simulink model "BLAC_MotorCtrl_Math"  (R2025b)
settings: Solver=FixedStepDiscrete  StartTime=0.0  StopTime=5  FixedStep=MC_Sim_BaseStep  RelTol=1e-3  EnableMultiTasking=on
values from neighbouring files (symbols this model uses):
  MC_Hardware_Chip_ADCResultBit = 0.0    [MotorControlDataDictionary_Math.sldd]
  MC_Hardware_Chip_ADCVoltageMax = 1.0    [MotorControlDataDictionary_Math.sldd]
  MC_Hardware_Chip_ADCVoltageRefence = 0.0    [MotorControlDataDictionary_Math.sldd]
  MC_Hardware_Chip_CSAGain = 1.0    [MotorControlDataDictionary_Math.sldd]
  MC_Sim_BaseStep = 2.5E-8    [MotorControlDataDictionary_Math.sldd]
  MC_Sim_HFTStep = 6.6675E-5    [MotorControlDataDictionary_Math.sldd]
undefined symbols (not defined in the file or in its folder): MC_MOS_DeadTime, MC_Motor_Phi, MC_Motor_Rotor_Pn, MC_Motor_Stator_Ld, MC_Motor_Stator_Lq, MC_Motor_Stator_Rs, MC_Param_CurrentPI_Ki, MC_Param_CurrentPI_Kp, MC_Param_CurrentPI_UdInteMax, MC_Param_CurrentPI_UdInteMin, MC_Param_CurrentPI_UdMax, MC_Param_CurrentPI_UdMin, MC_Param_CurrentPI_UqInteMax, MC_Param_CurrentPI_UqInteMin, MC_Param_CurrentPI_UqMax, MC_Param_CurrentPI_UqMin, MC_Param_Flux_Gamma, MC_Param_Flux_Lalpha, MC_Param_Flux_Lbeta, MC_Param_Flux_Ralpha, MC_Param_Flux_Rbeta, MC_Param_Luen_BEMFalpha, MC_Param_Luen_BEMFbeta, MC_Param_Luen_BEMFErr, MC_Param_Luen_Currentalpha, MC_Param_Luen_Currentbeta, MC_Param_Luen_CurrentErr, MC_Param_Luen_PLL_Ki, MC_Param_Luen_PLL_Kp, MC_Param_Luen_Voltagealpha, MC_Param_Luen_Voltagebeta, MC_Param_PhasetoReal, MC_Param_SMO_CoffA, MC_Param_SMO_CoffB, MC_Param_SpeedtoTheta, MC_Param_SVPWM_DutyMax, MC_Param_SVPWM_DutyMin, MC_Param_SVPWM_SampleOffset1, MC_Param_SVPWM_SampleOffset2, MC_Param_SVPWM_SampleValid
libraries: simulink x31, nesl_utility x22, ee_lib x21, fl_lib x16, spsSeriesRLCBranchLib x2, spsVoltageMeasurementLib x2
(part 2 of 5)

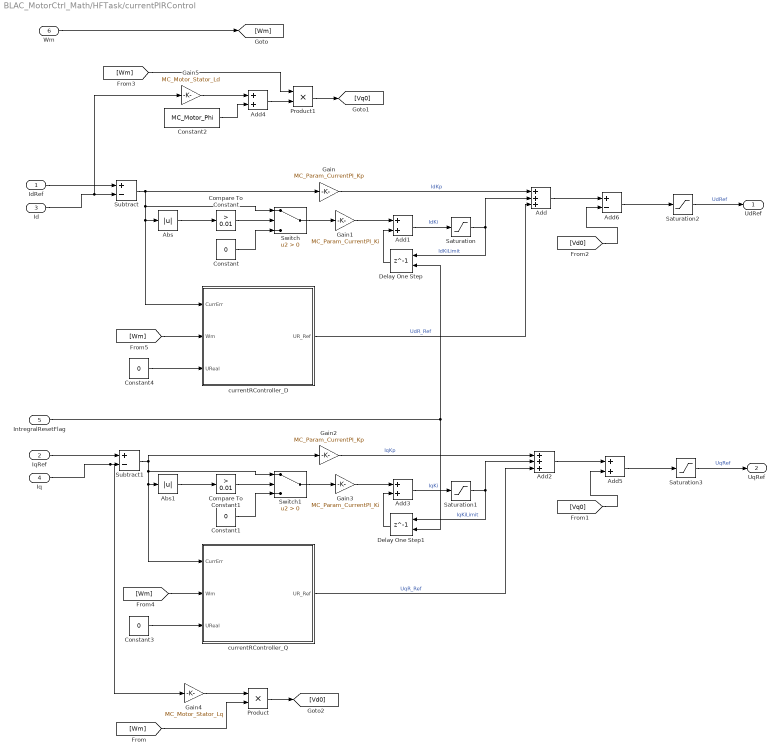
== system BLAC_MotorCtrl_Math/HFTask/currentPIRControl ==
  IdRef : Inport
  IqRef : Inport  Port=2
  Id : Inport  Port=3
  Iq : Inport  Port=4
  IntregralResetFlag : Inport  Port=5
  Wm : Inport  Port=6
  Abs : Abs  SaturateOnIntegerOverflow=off
  Abs1 : Abs  SaturateOnIntegerOverflow=off
  Add : Sum  Inputs=+++
  Add1 : Sum  OutDataTypeStr=single
  Add2 : Sum  Inputs=+++
  Add3 : Sum  OutDataTypeStr=single
  Add4 : Sum
  Add5 : Sum
  Add6 : Sum  Inputs=+-
  Compare To Constant : simulink/Logic and Bit Operations/Compare To Constant  relop=>  const=0.01  OutDataTypeStr=boolean
  Compare To Constant1 : simulink/Logic and Bit Operations/Compare To Constant  relop=>  const=0.01  OutDataTypeStr=boolean
  Constant{,1,3..4} (4 alike) : Constant  Value=0  OutDataTypeStr=single
  Constant2 : Constant  Value=MC_Motor_Phi  OutDataTypeStr=single
  Delay One Step : Delay  DelayLength=1  ExternalReset=Level
      settings: InputPortMap=u0,r5
  Delay One Step1 : Delay  DelayLength=1  ExternalReset=Level
      settings: InputPortMap=u0,r5
  Gain : Gain  Gain=MC_Param_CurrentPI_Kp  OutDataTypeStr=single
  Gain1 : Gain  Gain=MC_Param_CurrentPI_Ki  OutDataTypeStr=single
  Gain2 : Gain  Gain=MC_Param_CurrentPI_Kp  OutDataTypeStr=single
  Gain3 : Gain  Gain=MC_Param_CurrentPI_Ki  OutDataTypeStr=single
  Gain4 : Gain  Gain=MC_Motor_Stator_Lq
  Gain5 : Gain  Gain=MC_Motor_Stator_Ld
  Product : Product
  Product1 : Product
  Saturation : Saturate  UpperLimit=MC_Param_CurrentPI_UdInteMax  LowerLimit=MC_Param_CurrentPI_UdInteMin
  Saturation1 : Saturate  UpperLimit=MC_Param_CurrentPI_UqInteMax  LowerLimit=MC_Param_CurrentPI_UqInteMin
  Saturation2 : Saturate  UpperLimit=MC_Param_CurrentPI_UdMax  LowerLimit=MC_Param_CurrentPI_UdMin
  Saturation3 : Saturate  UpperLimit=MC_Param_CurrentPI_UqMax  LowerLimit=MC_Param_CurrentPI_UqMin
  Subtract : Sum  Inputs=+-
  Subtract1 : Sum  Inputs=+-
  Switch : Switch  Criteria=u2 > Threshold  SaturateOnIntegerOverflow=off  InputSameDT=off
  Switch1 : Switch  Criteria=u2 > Threshold  SaturateOnIntegerOverflow=off  InputSameDT=off
  currentRController_D : Subsystem
  currentRController_Q : Subsystem
  UdRef : Outport
  UqRef : Outport  Port=2
  wires:
  Subtract1/1 -> Gain2/1, currentRController_Q/1(CurrErr), Abs1/1, Switch1/1
  Wm/1 -> [Wm]
  [Wm] -> Product1/1
  Saturation3/1 -> UqRef/1  "UqRef"
  Saturation2/1 -> UdRef/1  "UdRef"
  [Vd0] -> Add6/2
  Add6/1 -> Saturation2/1
  Add/1 -> Add6/1
  [Vq0] -> Add5/2
  Add2/1 -> Add5/1
  Product/1 -> [Vd0]
  Product1/1 -> [Vq0]
  Constant2/1 -> Add4/2
  Add4/1 -> Product1/2
  Gain5/1 -> Add4/1
  [Wm] -> Product/2
  Id/1 -> Subtract/2, Gain5/1
  Gain4/1 -> Product/1
  Switch1/1 -> Gain3/1
  Abs1/1 -> Compare To Constant1/1
  Compare To Constant1/1 -> Switch1/2
  Constant1/1 -> Switch1/3
  Constant/1 -> Switch/3
  Compare To Constant/1 -> Switch/2
  Switch/1 -> Gain1/1
  Add5/1 -> Saturation3/1
  IntregralResetFlag/1 -> Delay One Step1/2, Delay One Step/2
  IqRef/1 -> Subtract1/1
  Iq/1 -> Gain4/1, Subtract1/2
  Gain2/1 -> Add2/1  "IqKp"
  Gain3/1 -> Add3/1
  Delay One Step1/1 -> Add3/2
  Add3/1 -> Saturation1/1  "IqKi"
  Saturation1/1 -> Add2/2, Delay One Step1/1  "IqKiLimit"
  Saturation/1 -> Delay One Step/1, Add/2  "IdKiLimit"
  Add1/1 -> Saturation/1  "IdKi"
  Delay One Step/1 -> Add1/2
  Gain1/1 -> Add1/1
  Abs/1 -> Compare To Constant/1
  Gain/1 -> Add/1  "IdKp"
  Subtract/1 -> currentRController_D/1(CurrErr), Abs/1, Switch/1, Gain/1
  IdRef/1 -> Subtract/1
  currentRController_D/1(UR_Ref) -> Add/3  "UdR_Ref"
  currentRController_Q/1(UR_Ref) -> Add2/3  "UqR_Ref"
  [Wm] -> currentRController_Q/2(Wm)
  Constant3/1 -> currentRController_Q/3(UReal)
  Constant4/1 -> currentRController_D/3(UReal)
  [Wm] -> currentRController_D/2(Wm)

== system BLAC_MotorCtrl_Math/HFTask/fluxobservor ==
  Valpha : Inport
  Vbeta : Inport  Port=2
  Ialpha : Inport  Port=3
  Ibeta : Inport  Port=4
  getFlux : Subsystem
  getSpeedandTheta : Subsystem
  Speed : Outport
  Theta : Outport  Port=2
  wires:
  getSpeedandTheta/2(Theta) -> Theta/1
  getSpeedandTheta/1(Speed) -> Speed/1
  getFlux/2(Phibeta) -> getSpeedandTheta/2(Phibeta)
  getFlux/1(Phialpha) -> getSpeedandTheta/1(Phialpha)
  Ibeta/1 -> getFlux/4(Ibeta)
  Ialpha/1 -> getFlux/3(Ialpha)
  Vbeta/1 -> getFlux/2(Vbeta)
  Valpha/1 -> getFlux/1(Valpha)

== system BLAC_MotorCtrl_Math/HFTask/getCurrentPredict ==
  note: 开发日志：
      | 2025.03.26:
      | 1、完成两节拍的电流预测
      | 2025.03.27：
      | 1、采用延时2个周期的采样电流和延时1个周期的设定电压进行延时1个周期的电机电流预测
  Ud1 : Inport
  Id : Inport  Port=2
  Uq1 : Inport  Port=3
  Iq : Inport  Port=4
  Wm : Inport  Port=5
  Add : Sum  Inputs=+++
  Add1 : Sum  Inputs=++-
  Add2 : Sum
  Constant : Constant  Value=MC_Motor_Phi  OutDataTypeStr=single
  Gain1 : Gain  Gain=MC_Sim_HFTStep/MC_Motor_Stator_Lq
  Gain4 : Gain  Gain=MC_Sim_HFTStep/MC_Motor_Stator_Ld
  Gain5 : Gain  Gain=1-(MC_Sim_HFTStep*MC_Motor_Stator_Rs/MC_Motor_Stator_Ld)
  Gain6 : Gain  Gain=MC_Sim_HFTStep/MC_Motor_Stator_Lq
  Gain7 : Gain  Gain=1-(MC_Sim_HFTStep*MC_Motor_Stator_Rs/MC_Motor_Stator_Lq)
  Gain8 : Gain  Gain=MC_Sim_HFTStep*MC_Motor_Stator_Ld/MC_Motor_Stator_Lq
  Gain9 : Gain  Gain=(MC_Sim_HFTStep*MC_Motor_Stator_Lq/MC_Motor_Stator_Ld)
  Product : Product
  Product1 : Product
  Id_Pre : Outport
  Iq_Pre : Outport  Port=2
  wires:
  [Iq] -> Gain7/1
  [Wm] -> Product1/1
  Iq/1 -> [Iq]
  Gain4/1 -> Add/1  "Ud_Id1"
  [Iq] -> Gain9/1
  [Uq1] -> Gain6/1
  Gain9/1 -> Product/1
  Constant/1 -> Gain1/1
  Product/1 -> Add/3  "Iq_Id1"
  [Ud1] -> Gain4/1
  Gain6/1 -> Add1/1  "Uq_Iq1"
  Gain7/1 -> Add1/2  "Iq_Iq1"
  Gain5/1 -> Add/2  "Id_Id1"
  [Id] -> Gain8/1
  Product1/1 -> Add1/3  "Id_Iq1"
  Gain8/1 -> Add2/1
  [Wm] -> Product/2
  Id/1 -> [Id]
  Add2/1 -> Product1/2
  [Id] -> Gain5/1
  Wm/1 -> [Wm]
  Gain1/1 -> Add2/2
  Add/1 -> Id_Pre/1  "Id1"
  Add1/1 -> Iq_Pre/1  "Iq1"
  Ud1/1 -> [Ud1]
  Uq1/1 -> [Uq1]

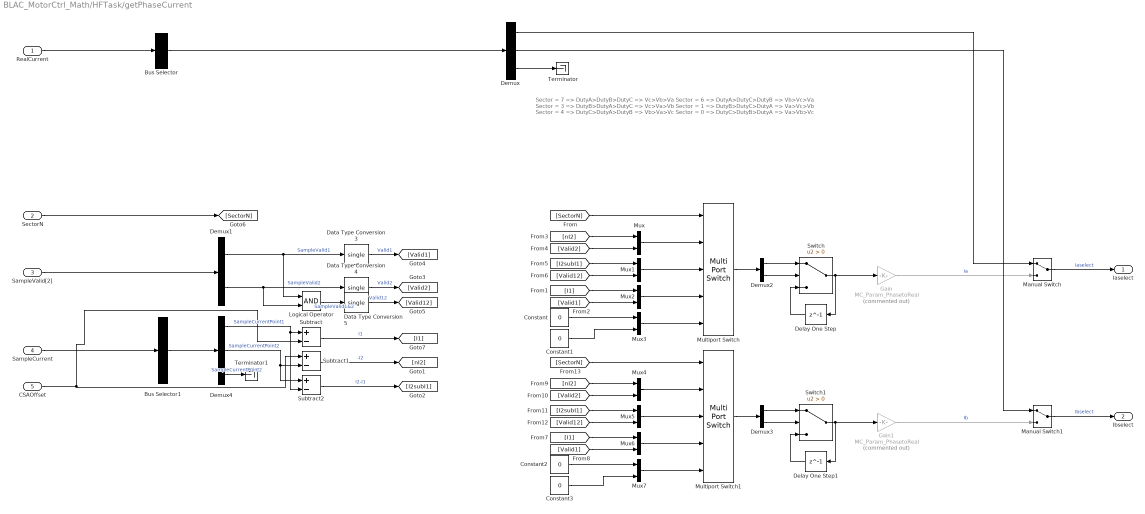
== system BLAC_MotorCtrl_Math/HFTask/getPhaseCurrent ==
  note: Sector = 7 => DutyA>DutyB>DutyC => Vc>Vb>Va
      | Sector = 6 => DutyA>DutyC>DutyB => Vb>Vc>Va
      | Sector = 3 => DutyB>DutyA>DutyC => Vc>Va>Vb
      | Sector = 1 => DutyB>DutyC>DutyA => Va>Vc>Vb
      | Sector = 4 => DutyC>DutyA>DutyB => Vb>Va>Vc
      | Sector = 0 => DutyC>DutyB>DutyA => Va>Vb>Vc
  RealCurrent : Inport
  SectorN : Inport  Port=2
  SampleValid[2] : Inport  Port=3
  SampleCurrent : Inport  Port=4
  CSAOffset : Inport  Port=5
  Bus Selector : BusSelector  OutputSignals=Iabc  OutputAsBus=on
  Bus Selector1 : BusSelector  OutputSignals=Iabc  OutputAsBus=on
  Constant{,1..3} (4 alike) : Constant  Value=0  OutDataTypeStr=single
  Data Type Conversion3 : DataTypeConversion  OutDataTypeStr=single  RndMeth=Simplest  SaturateOnIntegerOverflow=off
  Data Type Conversion4 : DataTypeConversion  OutDataTypeStr=single  RndMeth=Simplest  SaturateOnIntegerOverflow=off
  Data Type Conversion5 : DataTypeConversion  OutDataTypeStr=single  RndMeth=Simplest  SaturateOnIntegerOverflow=off
  Delay One Step : Delay  DelayLength=1
  Delay One Step1 : Delay  DelayLength=1
  Demux : Demux  Outputs=3
  Demux1 : Demux  Outputs=2
  Demux2 : Demux  Outputs=2
  Demux3 : Demux  Outputs=2
  Demux4 : Demux  Outputs=3
  Gain : Gain  Commented=on  Gain=MC_Param_PhasetoReal
  Gain1 : Gain  Commented=on  Gain=MC_Param_PhasetoReal
  Logical Operator : Logic  AllPortsSameDT=off  OutDataTypeStr=boolean
  Manual Switch : ManualSwitch
  Manual Switch1 : ManualSwitch
  Multiport Switch : MultiPortSwitch  DataPortOrder=Specify indices  DataPortIndices={[7,6],[3,4],[0,1]}  DataPortForDefault=Additional data port  SaturateOnIntegerOverflow=off  InputSameDT=off
  Multiport Switch1 : MultiPortSwitch  DataPortOrder=Specify indices  DataPortIndices={[3,1],[7,0],[6,4]}  DataPortForDefault=Additional data port  SaturateOnIntegerOverflow=off  InputSameDT=off
  Mux{,1..7} (8 alike) : Mux  Inputs=2
  Subtract : Sum  Inputs=+-
  Subtract1 : Sum  Inputs=+-
  Subtract2 : Sum  Inputs=+-
  Switch : Switch  Criteria=u2 > Threshold  SaturateOnIntegerOverflow=off  InputSameDT=off
  Switch1 : Switch  Criteria=u2 > Threshold  SaturateOnIntegerOverflow=off  InputSameDT=off
  Terminator : Terminator
  Terminator1 : Terminator
  Iaselect : Outport
  Ibselect : Outport  Port=2
  wires:
  RealCurrent/1 -> Bus Selector/1
  Bus Selector/1 -> Demux/1
  Manual Switch/1 -> Iaselect/1  "Iaselect"
  Demux/3 -> Terminator/1
  Manual Switch1/1 -> Ibselect/1  "Ibselect"
  Multiport Switch1/1 -> Demux3/1
  Demux3/2 -> Switch1/2
  Demux3/1 -> Switch1/1
  Switch1/1 -> Delay One Step1/1, Gain1/1
  Delay One Step1/1 -> Switch1/3
  Gain1/1 -> Manual Switch1/2  "Ib"
  Gain/1 -> Manual Switch/2  "Ia"
  Delay One Step/1 -> Switch/3
  Switch/1 -> Gain/1, Delay One Step/1
  Demux2/1 -> Switch/1
  Demux2/2 -> Switch/2
  Multiport Switch/1 -> Demux2/1
  [SectorN] -> Multiport Switch1/1
  Mux4/1 -> Multiport Switch1/2
  Mux5/1 -> Multiport Switch1/3
  Mux6/1 -> Multiport Switch1/4
  [I1] -> Mux6/1
  [Valid1] -> Mux6/2
  [nI2] -> Mux4/1
  [Valid2] -> Mux4/2
  [Valid12] -> Mux5/2
  [I2subI1] -> Mux5/1
  Mux7/1 -> Multiport Switch1/5
  Constant2/1 -> Mux7/1
  Constant3/1 -> Mux7/2
  Subtract/1 -> [I1]  "I1"
  Subtract1/1 -> [nI2]  "-I2"
  Data Type Conversion5/1 -> [Valid12]  "Valid12"
  Data Type Conversion4/1 -> [Valid2]  "Valid2"
  Data Type Conversion3/1 -> [Valid1]  "Valid1"
  Subtract2/1 -> [I2subI1]  "I2-I1"
  Constant1/1 -> Mux3/2
  Constant/1 -> Mux3/1
  Mux3/1 -> Multiport Switch/5
  [I2subI1] -> Mux1/1
  [Valid12] -> Mux1/2
  [Valid2] -> Mux/2
  [nI2] -> Mux/1
  [Valid1] -> Mux2/2
  [I1] -> Mux2/1
  [SectorN] -> Multiport Switch/1
  SectorN/1 -> [SectorN]
  Mux2/1 -> Multiport Switch/4
  Mux1/1 -> Multiport Switch/3
  Mux/1 -> Multiport Switch/2
  Logical Operator/1 -> Data Type Conversion5/1  "SampleValid1&2"
  Demux1/2 -> Data Type Conversion4/1, Logical Operator/2  "SampleValid2"
  Demux1/1 -> Data Type Conversion3/1, Logical Operator/1  "SampleValid1"
  SampleValid[2]/1 -> Demux1/1
  Demux4/2 -> Subtract2/1, Subtract1/2  "SampleCurrentPoint2"
  CSAOffset/1 -> Subtract1/1, Subtract/2
  Demux4/1 -> Subtract2/2, Subtract/1  "SampleCurrentPoint1"
  Bus Selector1/1 -> Demux4/1
  SampleCurrent/1 -> Bus Selector1/1
  Demux/1 -> Manual Switch/1
  Demux/2 -> Manual Switch1/1
  Demux4/3 -> Terminator1/1  "SampleCurrentPoint2"

== system BLAC_MotorCtrl_Math/HFTask/getSinCos ==
  Theta : Inport
  Sin : Trigonometry
  Sin1 : Trigonometry  Operator=cos
  SinTheta : Outport
  CosTheta : Outport  Port=2
  wires:
  Theta/1 -> Sin1/1, Sin/1
  Sin/1 -> SinTheta/1
  Sin1/1 -> CosTheta/1

== system BLAC_MotorCtrl_Math/HFTask/invParkTransform ==
  Ud : Inport
  Uq : Inport  Port=2
  SinTheta : Inport  Port=3
  CosTheta : Inport  Port=4
  Add : Sum
  Product{,1..3} (4 alike) : Product
  Subtract : Sum  Inputs=+-
  Ualpha : Outport
  Ubeta : Outport  Port=2
  wires:
  Uq/1 -> Product3/1, Product1/1
  Subtract/1 -> Ualpha/1  "Ualpha"
  CosTheta/1 -> Product/2, Product3/2
  SinTheta/1 -> Product2/2, Product1/2
  Product/1 -> Subtract/1
  Product1/1 -> Subtract/2
  Ud/1 -> Product/1, Product2/1
  Product2/1 -> Add/1
  Product3/1 -> Add/2
  Add/1 -> Ubeta/1  "Ubeta"

== system BLAC_MotorCtrl_Math/HFTask/karmalObservor ==
  In1 : Inport
  Out1 : Outport
  wires:
  In1/1 -> Out1/1

== system BLAC_MotorCtrl_Math/HFTask/scvmobservor ==
  Vd : Inport
  Vq : Inport  Port=2
  Id : Inport  Port=3
  Iq : Inport  Port=4
  getW : Subsystem
  wires:
  Vd/1 -> getW/1(Vd)
  Vq/1 -> getW/2(Vq)
  Id/1 -> getW/3(Id)
  Iq/1 -> getW/4(Iq)

== system BLAC_MotorCtrl_Math/HFTask/smo ==
  Valpha : Inport
  Vbeta : Inport  Port=2
  Ialpha : Inport  Port=3
  Ibeta : Inport  Port=4
  getE : Subsystem
  getSpeedandTheta : Subsystem
  Speed : Outport
  Theta : Outport  Port=2
  wires:
  Valpha/1 -> getE/1(Valpha)
  Vbeta/1 -> getE/2(Vbeta)
  Ialpha/1 -> getE/3(Ialpha)
  Ibeta/1 -> getE/4(Ibeta)
  getE/1(Ealpha) -> getSpeedandTheta/1(Ealpha)
  getE/2(Ebeta) -> getSpeedandTheta/2(Ebeta)
  getSpeedandTheta/1(Speed) -> Speed/1
  getSpeedandTheta/2(Theta) -> Theta/1

== system BLAC_MotorCtrl_Math/HFTask/svpwm ==
  Valpha : Inport
  Vbeta : Inport  Port=2
  Vdc : Inport  Port=3
  Ia : Inport  Port=4
  Ib : Inport  Port=5
  PhaseShortEnableFlag : Inport  Port=6
  Terminator : Terminator
  getVoltageExchange : Subsystem
  setDTCompelte : Subsystem
  setPhaseandSample_ORS_Double : Subsystem
  setPhaseandSample_ORS_Double1 : Subsystem  Commented=on
  DutySVPWM : Outport
  SamplePoint : Outport  Port=2
  SampleValid : Outport  Port=3
  SectorN : Outport  Port=4
  wires:
  Valpha/1 -> getVoltageExchange/1(Valpha)
  Vbeta/1 -> getVoltageExchange/2(Vbeta)
  Vdc/1 -> getVoltageExchange/3(Vdc)
  getVoltageExchange/1(Va) -> setDTCompelte/1(Va)
  getVoltageExchange/2(Vb) -> setDTCompelte/2(Vb)
  getVoltageExchange/3(Vc) -> setDTCompelte/3(Vc)
  getVoltageExchange/4(Vmed) -> setDTCompelte/4(Vmed)
  Ia/1 -> setDTCompelte/5(Ia)
  Ib/1 -> setDTCompelte/6(ib)
  setDTCompelte/1(SectorN) -> SectorN/1, setPhaseandSample_ORS_Double/1(SectorN)
  setDTCompelte/2(DutyLMS) -> setPhaseandSample_ORS_Double/2(DutyLMS)
  setPhaseandSample_ORS_Double/1(DutySVPWM) -> DutySVPWM/1
  setPhaseandSample_ORS_Double/2(SamplePoint) -> SamplePoint/1
  setPhaseandSample_ORS_Double/3(SampleValid) -> SampleValid/1
  PhaseShortEnableFlag/1 -> Terminator/1

== system BLAC_MotorCtrl_Math/HFTask/voltageLimit ==
  UdRef : Inport
  UqRef : Inport  Port=2
  Umax : Inport  Port=3
  Add : Sum
  Compare To Constant : simulink/Logic and Bit Operations/Compare To Constant  relop=<=  const=0  OutDataTypeStr=boolean
  Compare To Constant1 : simulink/Logic and Bit Operations/Compare To Constant  relop=>=  const=0  OutDataTypeStr=boolean
  Constant : Constant  Value=0  OutDataTypeStr=single
  Gain : Gain  Gain=-1
  Gain1 : Gain  Gain=-1
  Product : Product
  Saturation Dynamic : simulink/Discontinuities/Saturation Dynamic  OutMin=[]  OutMax=[]  OutDataTypeStr=Inherit: Same as second input  OutDataType=fixdt(1, 16)  OutScaling=2^-10  DoSatur=off
  Sqrt : Sqrt
  Subtract : Sum  Inputs=+-
  Switch : Switch  Criteria=u2 > Threshold  SaturateOnIntegerOverflow=off  InputSameDT=off
  Switch1 : Switch  Criteria=u2 > Threshold  SaturateOnIntegerOverflow=off  InputSameDT=off
  Switch2 : Switch  Criteria=u2 > Threshold  SaturateOnIntegerOverflow=off  InputSameDT=off
  Ud : Outport
  Uq : Outport  Port=2
  wires:
  Add/1 -> Product/1
  Subtract/1 -> Product/2
  Product/1 -> Compare To Constant/1, Sqrt/1
  Compare To Constant/1 -> [UdOverFlow]
  Sqrt/1 -> Gain/1, Saturation Dynamic/1
  Gain/1 -> Saturation Dynamic/3
  UdRef/1 -> [UdRef]
  UqRef/1 -> [UqRef]
  Umax/1 -> [Umax]
  [Umax] -> Subtract/1, Add/1
  [UdRef] -> Add/2, Subtract/2
  [UqRef] -> Saturation Dynamic/2
  Saturation Dynamic/1 -> Switch/3
  [UdOverFlow] -> Switch/2
  Constant/1 -> Switch/1
  Switch/1 -> Uq/1  "UqLimit"
  Switch1/1 -> Ud/1  "UdLimit"
  Switch2/1 -> Switch1/1
  [UdRef] -> Compare To Constant1/1
  Compare To Constant1/1 -> Switch2/2
  [Umax] -> Gain1/1, Switch2/1
  Gain1/1 -> Switch2/3
  [UdOverFlow] -> Switch1/2
  [UdRef] -> Switch1/3

== system BLAC_MotorCtrl_Math/Hardware_Sim/ActoDC_Sim ==
  Diode{,1..3} (4 alike) : ee_lib/Semiconductors & Converters/Diode  ModelType=ee.enum.diode.modelType.pwl  TableType=ee.enum.diode.tableType.IfMat  IfMat=[.07, .12, .19, 1.75, 4.24, 7.32, 11.2; .16, .3, .72, 2.14, 5.02, 8.35, 13.12] A  VfMat=[.9, 1.15, 1.25, 1.5, 1.75, 2.17, 2.6, 2.85; .58, .68, .75, 1.1, 1.38, 1.77, 2.27, 2.7] V  TjVec=[25, 125] degC  VfVec=[.5, .7, .9, 1.3, 1.7, 2.1, 2.5] V  IfVec=[.1, .2, .5, 1, 2, 4, 7, 10] A  IrMat=[1e-06, 2e-06, 5e-06, 1e-05, 2.5e-05, 5e-05, .0001; 2e-06, 5e-06, 1e-05, 4e-05, 8e-05, .0002, .0005] A  VrMat=[10, 100, 200, 250, 300, 325, 350; 10, 70, 160, 220, 270, 300, 320] V  VrVec=[10, 20, 40, 50, 70, 80, 100] V  IrVec=[1e-06, 2e-06, 5e-06, 1e-05, 2e-05, 5e-05, .0001] A  Vf=0.6 V  Ron=0.3 Ohm  Goff=1e-8 S  prmExp=ee.enum.diode.expParam.useTwo  I12=[.0137, .545] A  V12=[.6, .7] V  RS=0 Ohm  Tmeas=298.15 K  IS=1e-12 A  ec=1  I1=0.0137 A  V1=0.6 V  N_series=1  N_parallel=1  ZenerEnable=false  Rz=0.3 Ohm  BV=inf V  C_param=ee.enum.diode.capParam.fixed  CJ=0 pF  CJ0=5 pF  Vvec=[.1, 10, 100] V  Cvec=[3.5, 1, .4] pF  VJ=1 V  Mgrad=0.5  FC=0.5  Q_param=ee.enum.diode.recoveryParam.off  iRM=-7.15 A  iF=4 A  didt=-750 A/us  trr_factor=3  trr=115 ns  Qrr=150 nA*s  Vr=-600 V  Ls=150 nH  Erec=0.03 J  TT=50 ns  tau=100 ns  T_param=ee.enum.diode.temperatureParam.off  Tdevice=298.15 K  I1_T2=0.245 A  V1_T2=0.5 V  IS_T2=1.25e-7 A  Tmeas2=125 degC  XTI_param=ee.enum.diode.xtiParam.pn  XTI=3  EG_param=ee.enum.diode.egapParam.material_si  EG=1.11 eV  dBVdT=0 V/K  enable_fault_input=simscape.enum.onoff.off  i_specify=off  i_priority=None  i=0 A  i_nominal_specify=off  i_nominal_value=1  i_nominal_unit=A  v_specify=off  v_priority=None  v=0 V  v_nominal_specify=off  v_nominal_value=1  v_nominal_unit=V  v_capacitor_specify=off  v_capacitor_priority=None  v_capacitor=0 V  v_capacitor_nominal_specify=off  v_capacitor_nominal_value=1  v_capacitor_nominal_unit=V  Qj_specify=off  Qj_priority=High  Qj=0 C  Qj_nominal_specify=off  Qj_nominal_value=1  Qj_nominal_unit=C  i_diode_specify=off  i_diode_priority=None  i_diode=0 A  i_diode_nominal_specify=off  i_diode_nominal_value=1  i_diode_nominal_unit=A  v_diode_specify=off  v_diode_priority=None  v_diode=0 V  v_diode_nominal_specify=off  v_diode_nominal_value=1  v_diode_nominal_unit=V  i_capacitor_specify=off  i_capacitor_priority=None  i_capacitor=0 A  i_capacitor_nominal_specify=off  i_capacitor_nominal_value=1  i_capacitor_nominal_unit=A  power_dissipated_specify=off  power_dissipated_priority=None  power_dissipated=0 W  power_dissipated_nominal_specify=off  power_dissipated_nominal_value=1  power_dissipated_nominal_unit=W  fidelity_level=ee.enum.diode.fidelity.includeChargeDyn  rec_loss_model=ee.enum.diode.reverseRecoveryModel.fixed  ErecVal=0 J  scaleWithIandV=true  ErecMat=zeros(2, 3) J  TjrecVec=[298.15, 398.15] K  IfrecVec=[.1, 1, 10] A  IrecVal=10 A  VrecVal=10 V  tFilter=1 / 1000 / 100 s  thermal_network_parameterization=ee.enum.thermalNetworkTopology.junctionCase  Rth=[0, 10] K/W  Rth_Cauer=[1, 3, 10] K/W  Rth_Foster=[.08, .14, .22, .16] K/W  thermal_mass_parameterization=ee.enum.thermalNetwork.timeconstant  thermal_mass=[0, 1] J/K  thermal_mass_Cauer=[.1, .3, 1] J/K  thermal_mass_Foster=[.001, .005, .05, .5] J/K  thermal_time_constant=[0, 10] s  thermal_time_constant_Cauer=[1, 3, 10] s  thermal_time_constant_Foster=[7e-05, .0007, .01, .08] s  thermal_mass_initial_temperatures=[25, 25] degC  thermal_mass_initial_temperatures_Cauer=[25, 25, 25] degC  junction_thermal_mass=0.01 J/K  Tvec_initial_Foster=[25, 25, 25, 25] degC  no_thermal_network=0  junction_temperature_specify=off  junction_temperature_priority=None  junction_temperature=25 degC  junction_temperature_nominal_specify=off  junction_temperature_nominal_value=1  junction_temperature_nominal_unit=degC
  Electrical Reference : fl_lib/Electrical/Electrical Elements/Electrical Reference
  Resistor : ee_lib/Passive/Resistor  R=1 Ohm  enable_R_tol=ee.enum.toleranceApplication.none  R_tol=5  tol_distribution=ee.enum.toleranceDistribution.uniform  nSigma=4  enable_operating_limits=ee.enum.enable.no  operating_limit_action=ee.enum.passive.reportOpLim.warn  power_rating=1 W  max_working_voltage=100 V  noise_mode=ee.enum.sources.noise.Disabled  Tdevice=25 degC  sample_time=1e-3 s  repeatability=ee.enum.ic.repeatability.notRepeatable  user_seed=0  auto_seed=4120988592  power_derating_T1=70 degC  power_derating_T2=155 degC  operating_temperature_range_vec=[-50, 150] degC  alpha=3.93e-3 1/K  Tmeas=25 degC  thermal_mass=100 J/K  temperature_specify=off  temperature_priority=High  temperature=298.15 K  temperature_nominal_specify=off  temperature_nominal_value=1  temperature_nominal_unit=K
  Voltage Source : ee_lib/Sources/Voltage Source  dc_voltage=0 V  ac_voltage=220*sqrt(3) V  ac_shift=0 rad  ac_frequency=50 Hz  noise_mode=ee.enum.sources.noise.Disabled  PSD=0 V^2/Hz  sample_time=1e-3 s  repeatability=ee.enum.sources.repeatability.NotRepeatable  user_seed=0  auto_seed=3437178441  i_specify=off  i_priority=None  i=0 A  i_nominal_specify=off  i_nominal_value=1  i_nominal_unit=A  v_specify=off  v_priority=None  v=0 V  v_nominal_specify=off  v_nominal_value=1  v_nominal_unit=V
  Vdc_H : PMIOPort  Side=Right
  Vdc_L : PMIOPort  Port=2  Side=Right
  Vac_H : PMIOPort  Port=3  Side=Right
  Vac_L : PMIOPort  Port=4  Side=Right
  GND : PMIOPort  Port=5  Side=Right
  connections:
  Diode1/LConn1 -- Diode3/RConn1 -- Voltage Source/RConn1 -- Vac_L/RConn1
  Diode2/LConn1 -- Diode3/LConn1 -- Resistor/LConn1 -- Vdc_L/RConn1
  Diode/RConn1 -- Vdc_H/RConn1 -- Diode1/RConn1
  Diode2/RConn1 -- Diode/LConn1 -- Voltage Source/LConn1 -- Vac_H/RConn1
  Resistor/RConn1 -- Electrical Reference/LConn1 -- GND/RConn1

== system BLAC_MotorCtrl_Math/Hardware_Sim/CurrentSample_Sim ==
  Current_Sample_Trigger : Inport
  ADCSample_Sim : Subsystem  Commented=on
  PS-Simulink Converter{1..4} (4 alike) : nesl_utility/PS-Simulink Converter  PhysicalDomain=network_engine_domain  SubClassName=ps_output  LeftPortType=input  RightPortType=output  PseudoPeriodic=off  Frequencies=[]  VectorFormat=inherit  Unit=inherit  AffineConversion=off
  PhaseCurrentSmaple : Subsystem  Variant=on  VariantControl=PhaseCurrentSmaple
  Resistor1 : ee_lib/Passive/Resistor  R=1 Ohm  enable_R_tol=ee.enum.toleranceApplication.none  R_tol=5  tol_distribution=ee.enum.toleranceDistribution.uniform  nSigma=4  enable_operating_limits=ee.enum.enable.no  operating_limit_action=ee.enum.passive.reportOpLim.warn  power_rating=1 W  max_working_voltage=100 V  noise_mode=ee.enum.sources.noise.Disabled  Tdevice=25 degC  sample_time=1e-3 s  repeatability=ee.enum.ic.repeatability.notRepeatable  user_seed=0  auto_seed=3933054132  power_derating_T1=70 degC  power_derating_T2=155 degC  operating_temperature_range_vec=[-50, 150] degC  alpha=3.93e-3 1/K  Tmeas=25 degC  thermal_mass=100 J/K  temperature_specify=off  temperature_priority=High  temperature=298.15 K  temperature_nominal_specify=off  temperature_nominal_value=1  temperature_nominal_unit=K
  Resistor2 : ee_lib/Passive/Resistor  R=1 Ohm  enable_R_tol=ee.enum.toleranceApplication.none  R_tol=5  tol_distribution=ee.enum.toleranceDistribution.uniform  nSigma=4  enable_operating_limits=ee.enum.enable.no  operating_limit_action=ee.enum.passive.reportOpLim.warn  power_rating=1 W  max_working_voltage=100 V  noise_mode=ee.enum.sources.noise.Disabled  Tdevice=25 degC  sample_time=1e-3 s  repeatability=ee.enum.ic.repeatability.notRepeatable  user_seed=0  auto_seed=3402504572  power_derating_T1=70 degC  power_derating_T2=155 degC  operating_temperature_range_vec=[-50, 150] degC  alpha=3.93e-3 1/K  Tmeas=25 degC  thermal_mass=100 J/K  temperature_specify=off  temperature_priority=High  temperature=298.15 K  temperature_nominal_specify=off  temperature_nominal_value=1  temperature_nominal_unit=K
  Resistor3 : ee_lib/Passive/Resistor  R=1 Ohm  enable_R_tol=ee.enum.toleranceApplication.none  R_tol=5  tol_distribution=ee.enum.toleranceDistribution.uniform  nSigma=4  enable_operating_limits=ee.enum.enable.no  operating_limit_action=ee.enum.passive.reportOpLim.warn  power_rating=1 W  max_working_voltage=100 V  noise_mode=ee.enum.sources.noise.Disabled  Tdevice=25 degC  sample_time=1e-3 s  repeatability=ee.enum.ic.repeatability.notRepeatable  user_seed=0  auto_seed=1811450916  power_derating_T1=70 degC  power_derating_T2=155 degC  operating_temperature_range_vec=[-50, 150] degC  alpha=3.93e-3 1/K  Tmeas=25 degC  thermal_mass=100 J/K  temperature_specify=off  temperature_priority=High  temperature=298.15 K  temperature_nominal_specify=off  temperature_nominal_value=1  temperature_nominal_unit=K
  Resistor4 : ee_lib/Passive/Resistor  R=1 Ohm  enable_R_tol=ee.enum.toleranceApplication.none  R_tol=5  tol_distribution=ee.enum.toleranceDistribution.uniform  nSigma=4  enable_operating_limits=ee.enum.enable.no  operating_limit_action=ee.enum.passive.reportOpLim.warn  power_rating=1 W  max_working_voltage=100 V  noise_mode=ee.enum.sources.noise.Disabled  Tdevice=25 degC  sample_time=1e-3 s  repeatability=ee.enum.ic.repeatability.notRepeatable  user_seed=0  auto_seed=153380492  power_derating_T1=70 degC  power_derating_T2=155 degC  operating_temperature_range_vec=[-50, 150] degC  alpha=3.93e-3 1/K  Tmeas=25 degC  thermal_mass=100 J/K  temperature_specify=off  temperature_priority=High  temperature=298.15 K  temperature_nominal_specify=off  temperature_nominal_value=1  temperature_nominal_unit=K
  Voltage Sensor{1..4} (4 alike) : fl_lib/Electrical/Electrical Sensors/Voltage Sensor
  AL : PMIOPort  Side=Left
  BL : PMIOPort  Port=2  Side=Left
  CL : PMIOPort  Port=3  Side=Left
  GND : PMIOPort  Port=4  Side=Right
  Current_Sample : Outport
  wires:
  Current_Sample_Trigger/1 -> PhaseCurrentSmaple/1(SampleTrigger)
  PhaseCurrentSmaple/1(CurrentSampleResult) -> Current_Sample/1
  PS-Simulink Converter1/1 -> PhaseCurrentSmaple/3(SRV_B)
  PS-Simulink Converter2/1 -> PhaseCurrentSmaple/4(SRV_A)
  PS-Simulink Converter3/1 -> PhaseCurrentSmaple/2(SRV_C)
  PS-Simulink Converter4/1 -> PhaseCurrentSmaple/5(ShuntV)
  connections:
  Voltage Sensor2/LConn1 -- Resistor3/LConn1 -- AL/RConn1
  PS-Simulink Converter2/LConn1 -- Voltage Sensor2/RConn1
  Resistor1/LConn1 -- Voltage Sensor1/LConn1 -- BL/RConn1
  PS-Simulink Converter1/LConn1 -- Voltage Sensor1/RConn1
  Voltage Sensor3/LConn1 -- Resistor2/LConn1 -- CL/RConn1
  Voltage Sensor3/RConn2 -- Resistor2/RConn1
  PS-Simulink Converter3/LConn1 -- Voltage Sensor3/RConn1
  Voltage Sensor2/RConn2 -- Resistor3/RConn1
  PS-Simulink Converter4/LConn1 -- Voltage Sensor4/RConn1
  Voltage Sensor4/RConn2 -- Resistor4/RConn1 -- GND/RConn1
  Voltage Sensor4/LConn1 -- Resistor4/LConn1 -- Resistor1/RConn1 -- Voltage Sensor1/RConn2

== system BLAC_MotorCtrl_Math/Hardware_Sim/DrivePWM_Sim ==
  ClockCounter : Inport
  DrivePWM : Inport  Port=2
  Data Type Conversion{,1..5} (6 alike) : DataTypeConversion  OutDataTypeStr=double  RndMeth=Simplest  SaturateOnIntegerOverflow=off
  Demux : Demux  Outputs=6
  Mux : Mux  Inputs=2
  Mux1 : Mux  Inputs=2
  Mux2 : Mux  Inputs=2
  Relational Operator : RelationalOperator  Operator=>  OutDataTypeStr=boolean  RndMeth=Simplest  InputSameDT=off
  Relational Operator1 : RelationalOperator  Operator=>  OutDataTypeStr=boolean  RndMeth=Simplest  InputSameDT=off
  Relational Operator2 : RelationalOperator  Operator=>  OutDataTypeStr=boolean  RndMeth=Simplest  InputSameDT=off
  Relational Operator3 : RelationalOperator  Operator=<  OutDataTypeStr=boolean  RndMeth=Simplest  InputSameDT=off
  Relational Operator4 : RelationalOperator  Operator=<  OutDataTypeStr=boolean  RndMeth=Simplest  InputSameDT=off
  Relational Operator5 : RelationalOperator  Operator=<  OutDataTypeStr=boolean  RndMeth=Simplest  InputSameDT=off
  Drive_A : Outport
  Drive_B : Outport  Port=2
  Drive_C : Outport  Port=3
  wires:
  Relational Operator1/1 -> Data Type Conversion1/1
  DrivePWM/1 -> Demux/1
  Relational Operator2/1 -> Data Type Conversion3/1
  Relational Operator/1 -> Data Type Conversion/1
  Relational Operator3/1 -> Data Type Conversion2/1
  Relational Operator5/1 -> Data Type Conversion5/1
  Relational Operator4/1 -> Data Type Conversion4/1
  Demux/6 -> Relational Operator5/2
  Demux/5 -> Relational Operator4/2
  Demux/4 -> Relational Operator3/2
  Demux/3 -> Relational Operator2/2
  Demux/2 -> Relational Operator1/2
  Demux/1 -> Relational Operator/2
  ClockCounter/1 -> Relational Operator/1, Relational Operator1/1, Relational Operator2/1, Relational Operator3/1, Relational Operator4/1, Relational Operator5/1
  Data Type Conversion/1 -> Mux/1
  Mux/1 -> Drive_A/1
  Mux2/1 -> Drive_C/1
  Mux1/1 -> Drive_B/1
  Data Type Conversion1/1 -> Mux1/1
  Data Type Conversion3/1 -> Mux2/1
  Data Type Conversion2/1 -> Mux/2
  Data Type Conversion4/1 -> Mux1/2
  Data Type Conversion5/1 -> Mux2/2
